simulink model "AirManagementSystem"  (R2018b)
settings: Solver=ode4  StartTime=0.0  StopTime=14400  FixedStep=dt  RelTol=1e-3
values from neighbouring files (symbols this model uses):
  AirSourceMode = 2    [run_sim.m]
  dt = 0.01    [run_sim.m]    (also in sys_id_pipeline.m = mean(diff(Time_vec_full)))
  K31 = Result31.K_slope    [sys_id_pipeline.m]
  K32 = Result32.K_slope    [sys_id_pipeline.m]
  P_ref = GlobalParams.P_ref    [sys_id_pipeline.m]
  Patm = GlobalParams.Patm    [sys_id_pipeline.m]
  R_gas = GlobalParams.R    [sys_id_pipeline.m]
  T_ref = GlobalParams.T_ref    [sys_id_pipeline.m]
  Tau31 = 5    [sys_id_pipeline.m]
  Tau32 = 5    [sys_id_pipeline.m]
  Tp31 = Result31.Tp    [sys_id_pipeline.m]
  Tp32 = Result32.Tp    [sys_id_pipeline.m]
  V_vol = pi * (0.05)^2 * 5    (= 0.0392699081699)    [run_sim.m]
  X31_den = sys_X31.Denominator    [sys_id_value.m]
  X31_num = sys_X31.Numerator    [sys_id_value.m]
  X32_den = sys_X32.Denominator    [sys_id_value.m]
  X32_num = sys_X32.Numerator    [sys_id_value.m]
libraries: simulink x8
(part 1 of 2)
settings Model: Creator=ZhaoJiance  LastModifiedBy=ZhaoJiance

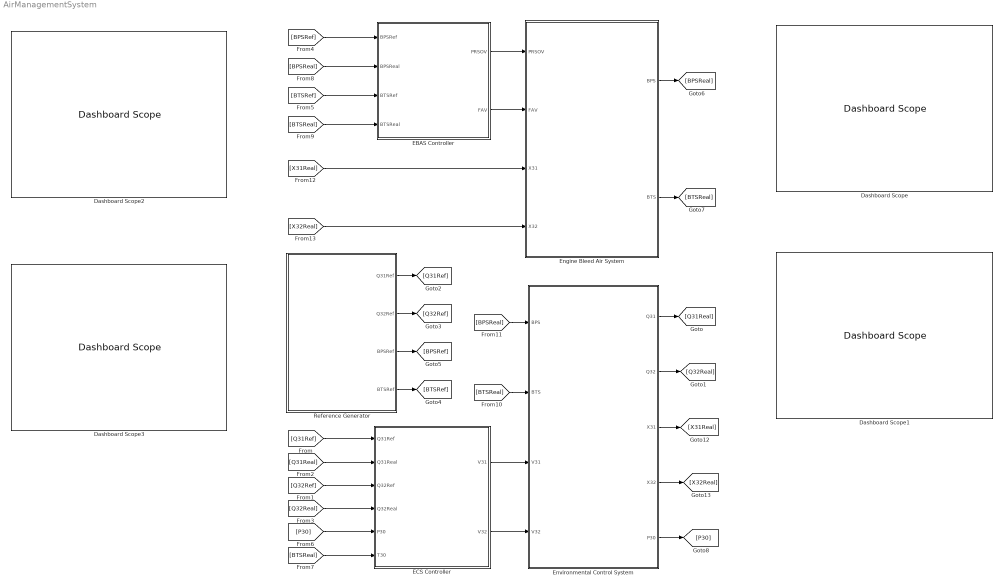
== system AirManagementSystem ==
  Dashboard Scope : DashboardScope  WebBlockId=509
  Dashboard Scope1 : DashboardScope  WebBlockId=510
  Dashboard Scope2 : DashboardScope  WebBlockId=511
  Dashboard Scope3 : DashboardScope  WebBlockId=512
  EBAS Controller : Subsystem  VariantControlMode=Label  Variant=on  VariantControl=Variant1  LabelModeActiveChoice=ASMC
  ECS Controller : Subsystem  VariantControlMode=Label  Variant=on  VariantControl=Variant1  LabelModeActiveChoice=Smith_PI_Controller
  Engine Bleed Air System : Subsystem
  Environmental Control System : Subsystem
  Reference Generator : Subsystem
  wires:
  Environmental Control System/1(Q31) -> [Q31Real]
  Environmental Control System/2(Q32) -> [Q32Real]
  [Q31Ref] -> ECS Controller/1("Q31Ref ")
  [Q31Real] -> ECS Controller/2("Q31Real ")
  [Q32Ref] -> ECS Controller/3("Q32Ref ")
  [Q32Real] -> ECS Controller/4("Q32Real ")
  [P30] -> ECS Controller/5("P30 ")
  [BTSReal] -> ECS Controller/6("T30 ")
  ECS Controller/1(" V31") -> Environmental Control System/3(V31)
  ECS Controller/2(" V32") -> Environmental Control System/4(V32)
  [BPSReal] -> Environmental Control System/1(BPS)
  [BTSReal] -> Environmental Control System/2(BTS)
  Environmental Control System/4(X32) -> [X32Real]
  Environmental Control System/3(X31) -> [X31Real]
  Reference Generator/3(BPSRef) -> [BPSRef]
  EBAS Controller/1(" PRSOV") -> Engine Bleed Air System/1(PRSOV)
  Reference Generator/2(Q32Ref) -> [Q32Ref]
  Engine Bleed Air System/2(BTS) -> [BTSReal]
  Reference Generator/1(Q31Ref) -> [Q31Ref]
  [BTSReal] -> EBAS Controller/4("BTSReal  ")
  [BPSRef] -> EBAS Controller/1("BPSRef  ")
  Engine Bleed Air System/1(BPS) -> [BPSReal]
  [BTSRef] -> EBAS Controller/3("BTSRef  ")
  EBAS Controller/2(" FAV") -> Engine Bleed Air System/2(FAV)
  [BPSReal] -> EBAS Controller/2("BPSReal ")
  Reference Generator/4(BTSRef) -> [BTSRef]
  [X31Real] -> Engine Bleed Air System/3(X31)
  [X32Real] -> Engine Bleed Air System/4(X32)
  Environmental Control System/5(P30) -> [P30]

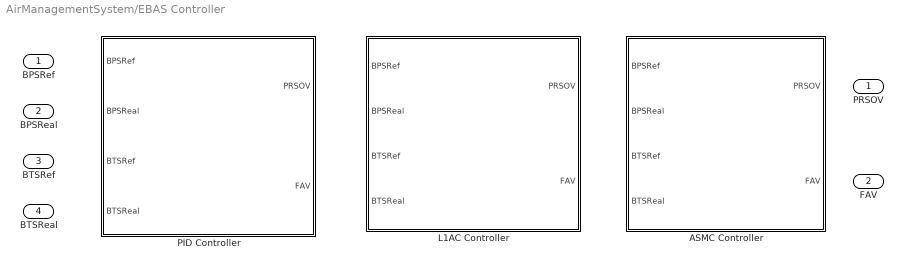
== system AirManagementSystem/EBAS Controller ==
  "BPSRef  " : Inport
  "BPSReal " : Inport  Port=2
  "BTSRef  " : Inport  Port=3
  "BTSReal  " : Inport  Port=4
  ASMC Controller : Subsystem  VariantControl=ASMC
  L1AC Controller : Subsystem  VariantControl=L1AC
  PID Controller : Subsystem  VariantControl=PID
  " PRSOV" : Outport
  " FAV" : Outport  Port=2

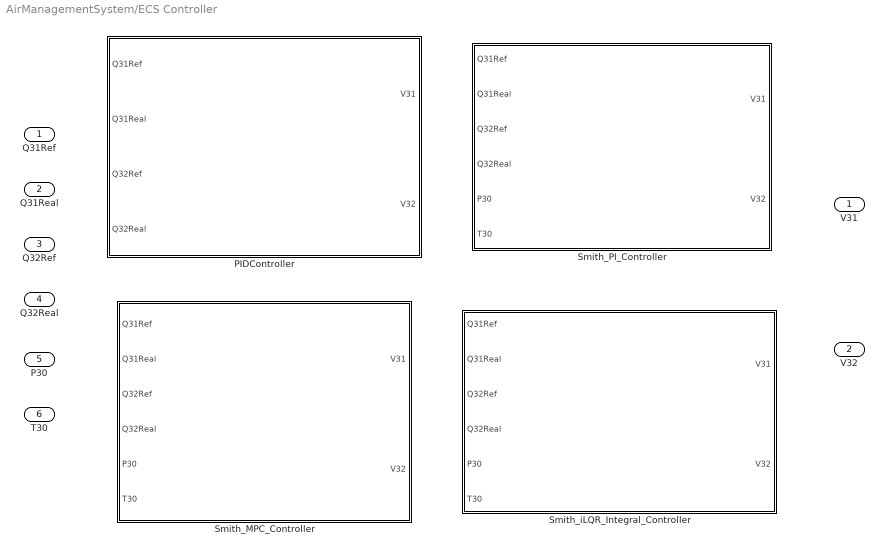
== system AirManagementSystem/ECS Controller ==
  "Q31Ref " : Inport
  "Q31Real " : Inport  Port=2
  "Q32Ref " : Inport  Port=3
  "Q32Real " : Inport  Port=4
  "P30 " : Inport  Port=5
  "T30 " : Inport  Port=6
  PIDController : Subsystem  VariantControl=PID
  Smith_MPC_Controller : Subsystem  VariantControl=Smith_MPC_Controller
  Smith_PI_Controller : Subsystem  VariantControl=Smith_PI_Controller
  Smith_iLQR_Integral_Controller : Subsystem  VariantControl=Variant
  " V31" : Outport
  " V32" : Outport  Port=2

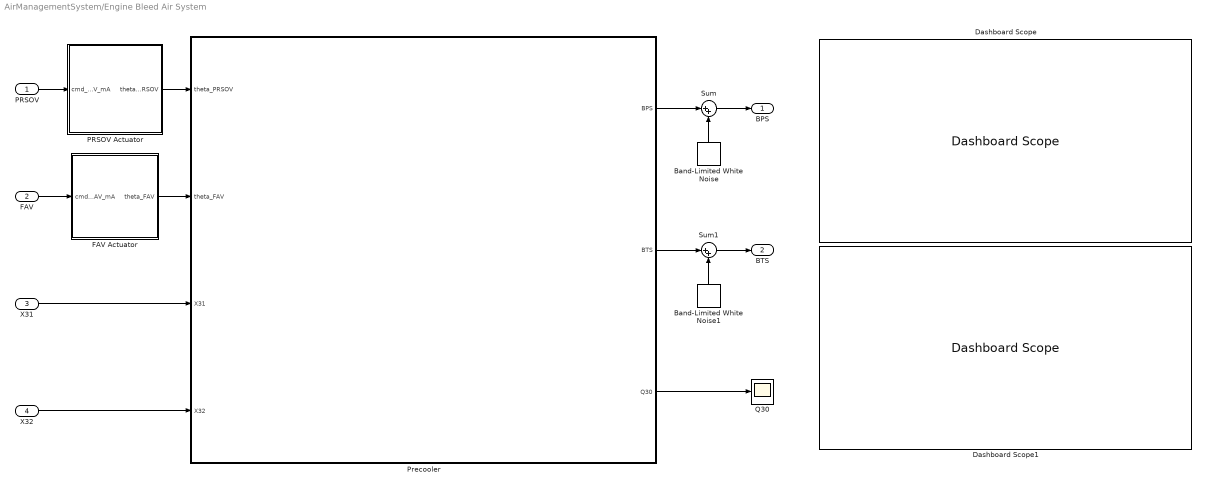
== system AirManagementSystem/Engine Bleed Air System ==
  PRSOV : Inport
  FAV : Inport  Port=2
  X31 : Inport  Port=3
  X32 : Inport  Port=4
  Band-Limited White Noise : simulink/Sources/Band-Limited White Noise  Cov=Knoise  Ts=dt  seed=[23341]
  Band-Limited White Noise1 : simulink/Sources/Band-Limited White Noise  Cov=Knoise  Ts=dt  seed=[23341]
  Dashboard Scope : DashboardScope  WebBlockId=669
  Dashboard Scope1 : DashboardScope  WebBlockId=670
  FAV Actuator : MATLAB Function  TreatAsAtomicUnit=on  SystemSampleTime=dt
  PRSOV Actuator : MATLAB Function  TreatAsAtomicUnit=on  SystemSampleTime=dt
  Precooler : Subsystem
      mask Display: image('C:\Users\ZhaoJiance\Documents\Github\AeroBleedSimulation\SysID\figure\Precooler.png');
  Q30 : Scope
  Sum : Sum  Inputs=|++
  Sum1 : Sum  Inputs=|++
  BPS : Outport
  BTS : Outport  Port=2
  wires:
  FAV/1 -> FAV Actuator/1(cmd_FAV_mA)
  PRSOV/1 -> PRSOV Actuator/1(cmd_PRSOV_mA)
  PRSOV Actuator/1(theta_PRSOV) -> Precooler/1(theta_PRSOV)
  FAV Actuator/1(theta_FAV) -> Precooler/2(theta_FAV)
  Precooler/3(Q30) -> Q30/1
  X31/1 -> Precooler/3(X31)
  X32/1 -> Precooler/4(X32)
  Sum/1 -> BPS/1
  Precooler/1(BPS) -> Sum/1
  Band-Limited White Noise/1 -> Sum/2
  Band-Limited White Noise1/1 -> Sum1/2
  Sum1/1 -> BTS/1
  Precooler/2(BTS) -> Sum1/1

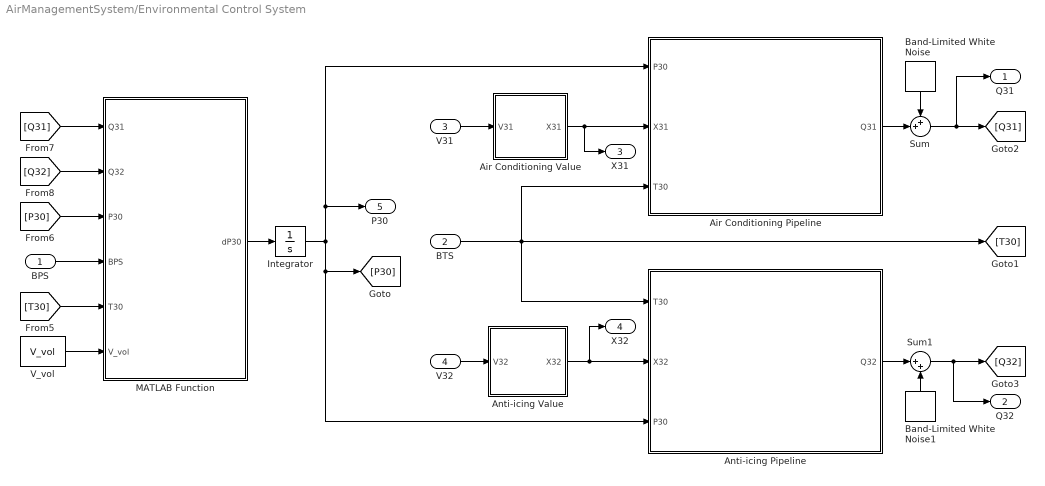
== system AirManagementSystem/Environmental Control System ==
  BPS : Inport
  BTS : Inport  Port=2
  V31 : Inport  Port=3
  V32 : Inport  Port=4
  Air Conditioning Pipeline : Subsystem
  Air Conditioning Value : Subsystem
  "Anti-icing Pipeline " : Subsystem
  Anti-icing Value : Subsystem
  Band-Limited White Noise : simulink/Sources/Band-Limited White Noise  Cov=Knoise  Ts=dt  seed=[23341]
  Band-Limited White Noise1 : simulink/Sources/Band-Limited White Noise  Cov=Knoise  Ts=dt  seed=[23341]
  Integrator : Integrator
  MATLAB Function : MATLAB Function  TreatAsAtomicUnit=on  SystemSampleTime=dt
  Sum : Sum  Inputs=++|
  Sum1 : Sum  Inputs=|++
  V_vol : Constant  Value=V_vol
  Q31 : Outport
  Q32 : Outport  Port=2
  X31 : Outport  Port=3
  X32 : Outport  Port=4
  P30 : Outport  Port=5
  wires:
  Air Conditioning Value/1(X31) -> X31/1, Air Conditioning Pipeline/2(X31)
  BPS/1 -> MATLAB Function/4(BPS)
  Integrator/1 -> Air Conditioning Pipeline/1(P30), P30/1, "Anti-icing Pipeline "/3(P30), [P30]
  Anti-icing Value/1(X32) -> X32/1, "Anti-icing Pipeline "/2(X32)
  V31/1 -> Air Conditioning Value/1(V31)
  MATLAB Function/1(dP30) -> Integrator/1
  [Q32] -> MATLAB Function/2(Q32)
  [Q31] -> MATLAB Function/1(Q31)
  V_vol/1 -> MATLAB Function/6(V_vol)
  [P30] -> MATLAB Function/3(P30)
  [T30] -> MATLAB Function/5(T30)
  V32/1 -> Anti-icing Value/1(V32)
  BTS/1 -> [T30], "Anti-icing Pipeline "/1(T30), Air Conditioning Pipeline/3(T30)
  Sum/1 -> [Q31], Q31/1
  Sum1/1 -> Q32/1, [Q32]
  "Anti-icing Pipeline "/1(Q32) -> Sum1/1
  Air Conditioning Pipeline/1(Q31) -> Sum/2
  Band-Limited White Noise/1 -> Sum/1
  Band-Limited White Noise1/1 -> Sum1/2

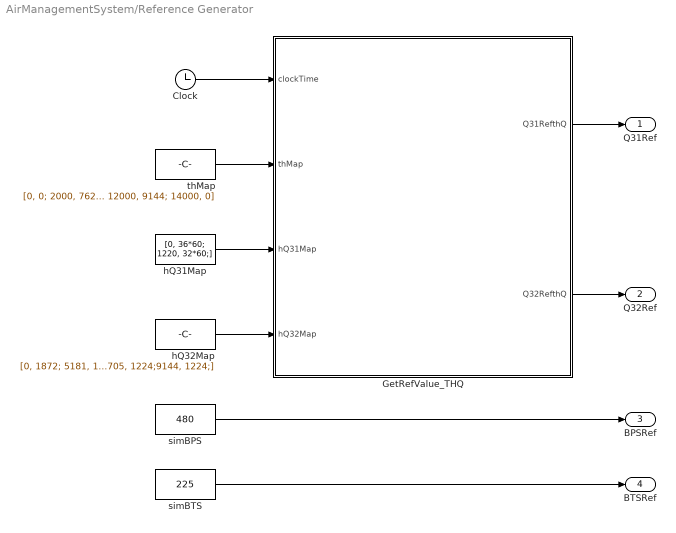
== system AirManagementSystem/Reference Generator ==
  Clock : Clock
  GetRefValue_THQ : MATLAB Function  TreatAsAtomicUnit=on  SystemSampleTime=dt
  hQ31Map : Constant  Value=[0, 36*60; 1220, 32*60;]
  hQ32Map : Constant  Value=[0, 1872; 5181, 1872; 6705, 1224;9144, 1224;]
  simBPS : Constant  Value=480
  simBTS : Constant  Value=225
  thMap : Constant  Value=[0, 0; 2000, 7620; 4000, 7620;6000, 12192; 8000, 12192; 10000, 9144; 12000, 9144; 14000, 0]
  Q31Ref : Outport
  Q32Ref : Outport  Port=2
  BPSRef : Outport  Port=3
  BTSRef : Outport  Port=4
  wires:
  Clock/1 -> GetRefValue_THQ/1(clockTime)
  thMap/1 -> GetRefValue_THQ/2(thMap)
  hQ31Map/1 -> GetRefValue_THQ/3(hQ31Map)
  GetRefValue_THQ/1(Q31RefthQ) -> Q31Ref/1
  hQ32Map/1 -> GetRefValue_THQ/4(hQ32Map)
  GetRefValue_THQ/2(Q32RefthQ) -> Q32Ref/1
  simBTS/1 -> BTSRef/1
  simBPS/1 -> BPSRef/1

== system AirManagementSystem/EBAS Controller/ASMC Controller ==
  "BPSRef  " : Inport
  "BPSReal " : Inport  Port=2
  "BTSRef  " : Inport  Port=3
  "BTSReal  " : Inport  Port=4
  ASMCController : MATLAB Function  TreatAsAtomicUnit=on  SystemSampleTime=dt
  " PRSOV" : Outport
  " FAV" : Outport  Port=2
  wires:
  ASMCController/1(PRSOV) -> " PRSOV"/1
  ASMCController/2(FAV) -> " FAV"/1
  "BPSRef  "/1 -> ASMCController/1(BPSRef)
  "BPSReal "/1 -> ASMCController/2(BPSReal)
  "BTSRef  "/1 -> ASMCController/3(BTSRef)
  "BTSReal  "/1 -> ASMCController/4(BTSReal)

== system AirManagementSystem/EBAS Controller/L1AC Controller ==
  "BPSRef  " : Inport
  "BPSReal " : Inport  Port=2
  "BTSRef  " : Inport  Port=3
  "BTSReal  " : Inport  Port=4
  FAV L1AC Controller : MATLAB Function  TreatAsAtomicUnit=on
  PRSOV L1AC Controller : MATLAB Function  TreatAsAtomicUnit=on
  " PRSOV" : Outport
  " FAV" : Outport  Port=2
  wires:
  FAV L1AC Controller/1(u_cmd) -> " FAV"/1
  PRSOV L1AC Controller/1(u_cmd) -> " PRSOV"/1
  "BPSRef  "/1 -> PRSOV L1AC Controller/1(Target)
  "BPSReal "/1 -> PRSOV L1AC Controller/2(Measured)
  "BTSReal  "/1 -> FAV L1AC Controller/2(Measured)
  "BTSRef  "/1 -> FAV L1AC Controller/1(Target)

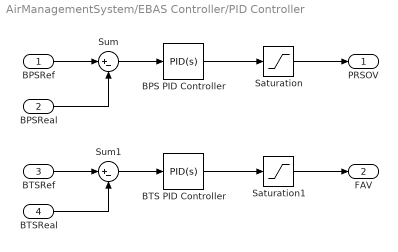
== system AirManagementSystem/EBAS Controller/PID Controller ==
  "BPSRef " : Inport
  BPSReal : Inport  Port=2
  "BTSRef " : Inport  Port=3
  "BTSReal " : Inport  Port=4
  BPS PID Controller : simulink/Continuous/PID Controller  Controller=PID  Form=Parallel  TimeDomain=Continuous-time  SampleTime=-1  IntegratorMethod=Forward Euler  FilterMethod=Forward Euler  ControllerParametersSource=internal  P=0.1  I=0.2  D=0.01  UseFilter=on  N=100  TunerSelectOption=Transfer Function Based (PID Tuner App)  InitialConditionSource=internal  InitialConditionForIntegrator=0  InitialConditionForFilter=0  DifferentiatorICPrevScaledInput=0  ExternalReset=none  TrackingMode=off  Kt=1  LimitOutput=off  UpperSaturationLimit=inf  LowerSaturationLimit=-inf  LinearizeAsGain=on  AntiWindupMode=none  Kb=1  POutMin=[]  POutMax=[]  IOutMin=[]  IOutMax=[]  DOutMin=[]  DOutMax=[]  NOutMin=[]  NOutMax=[]  SumOutMin=[]  SumOutMax=[]  SaturationOutMin=[]  SaturationOutMax=[]  PParamMin=[]  PParamMax=[]  IParamMin=[]  IParamMax=[]  DParamMin=[]  DParamMax=[]  NParamMin=[]  NParamMax=[]  KbParamMin=[]  KbParamMax=[]  KtParamMin=[]  KtParamMax=[]  KbOutMin=[]  KbOutMax=[]  KtOutMin=[]  KtOutMax=[]  IntegratorOutMin=[]  IntegratorOutMax=[]  FilterOutMin=[]  FilterOutMax=[]  SumI1OutMin=[]  SumI1OutMax=[]  SumI2OutMin=[]  SumI2OutMax=[]  SumI3OutMin=[]  SumI3OutMax=[]  SumI4OutMin=[]  SumI4OutMax=[]  SumDOutMin=[]  SumDOutMax=[]  DifferentiatorOutMin=[]  DifferentiatorOutMax=[]  FilterDiffOutCoefMin=[]  FilterDiffOutCoefMax=[]  ReciprocalOutMin=[]  ReciprocalOutMax=[]  SumDenOutMin=[]  SumDenOutMax=[]  SumNumOutMin=[]  SumNumOutMax=[]  DivideOutMin=[]  DivideOutMax=[]  IntegratorContinuousStateAttributes=''  IntegratorStateMustResolveToSignalObject=off  IntegratorRTWStateStorageClass=Auto  FilterContinuousStateAttributes=''  FilterStateMustResolveToSignalObject=off  FilterRTWStateStorageClass=Auto  ParallelPVariant=InternalParameters  IdealPVariant=Disabled  IVariant=InternalParameters  DVariant=InternalParameters  IntegratorVariant=Continuous  SatVariant=Disabled  AWVariant=Passthrough  PCopyVariant=Disabled  TRVariant=Disabled  FdbkBlocksVariant=Forward  IdealPFdbkVariant=Disabled  SatFdbkVariant=Disabled  DerivativeFilterVariant=ContFilter  NVariant=InternalParameters  NCopyVariant=Disabled  FilterICVariant=InternalICsFilter  IntegratorICVariant=InternalICs  ExternalResetVariant=Disabled  TRSumVariant=Passthrough  SumFdbkVariant=Disabled  SumVariant=Sum_PID
  BTS PID Controller : simulink/Continuous/PID Controller  Controller=PID  Form=Parallel  TimeDomain=Continuous-time  SampleTime=-1  IntegratorMethod=Forward Euler  FilterMethod=Forward Euler  ControllerParametersSource=internal  P=-0.1  I=-0.15  D=0  UseFilter=on  N=100  TunerSelectOption=Transfer Function Based (PID Tuner App)  InitialConditionSource=internal  InitialConditionForIntegrator=0  InitialConditionForFilter=0  DifferentiatorICPrevScaledInput=0  ExternalReset=none  TrackingMode=off  Kt=1  LimitOutput=off  UpperSaturationLimit=inf  LowerSaturationLimit=-inf  LinearizeAsGain=on  AntiWindupMode=none  Kb=1  POutMin=[]  POutMax=[]  IOutMin=[]  IOutMax=[]  DOutMin=[]  DOutMax=[]  NOutMin=[]  NOutMax=[]  SumOutMin=[]  SumOutMax=[]  SaturationOutMin=[]  SaturationOutMax=[]  PParamMin=[]  PParamMax=[]  IParamMin=[]  IParamMax=[]  DParamMin=[]  DParamMax=[]  NParamMin=[]  NParamMax=[]  KbParamMin=[]  KbParamMax=[]  KtParamMin=[]  KtParamMax=[]  KbOutMin=[]  KbOutMax=[]  KtOutMin=[]  KtOutMax=[]  IntegratorOutMin=[]  IntegratorOutMax=[]  FilterOutMin=[]  FilterOutMax=[]  SumI1OutMin=[]  SumI1OutMax=[]  SumI2OutMin=[]  SumI2OutMax=[]  SumI3OutMin=[]  SumI3OutMax=[]  SumI4OutMin=[]  SumI4OutMax=[]  SumDOutMin=[]  SumDOutMax=[]  DifferentiatorOutMin=[]  DifferentiatorOutMax=[]  FilterDiffOutCoefMin=[]  FilterDiffOutCoefMax=[]  ReciprocalOutMin=[]  ReciprocalOutMax=[]  SumDenOutMin=[]  SumDenOutMax=[]  SumNumOutMin=[]  SumNumOutMax=[]  DivideOutMin=[]  DivideOutMax=[]  IntegratorContinuousStateAttributes=''  IntegratorStateMustResolveToSignalObject=off  IntegratorRTWStateStorageClass=Auto  FilterContinuousStateAttributes=''  FilterStateMustResolveToSignalObject=off  FilterRTWStateStorageClass=Auto  ParallelPVariant=InternalParameters  IdealPVariant=Disabled  IVariant=InternalParameters  DVariant=InternalParameters  IntegratorVariant=Continuous  SatVariant=Disabled  AWVariant=Passthrough  PCopyVariant=Disabled  TRVariant=Disabled  FdbkBlocksVariant=Forward  IdealPFdbkVariant=Disabled  SatFdbkVariant=Disabled  DerivativeFilterVariant=ContFilter  NVariant=InternalParameters  NCopyVariant=Disabled  FilterICVariant=InternalICsFilter  IntegratorICVariant=InternalICs  ExternalResetVariant=Disabled  TRSumVariant=Passthrough  SumFdbkVariant=Disabled  SumVariant=Sum_PID
  Saturation : Saturate  UpperLimit=400  LowerLimit=0
  Saturation1 : Saturate  UpperLimit=350  LowerLimit=0
  Sum : Sum  Inputs=|+-
  Sum1 : Sum  Inputs=|+-
  PRSOV : Outport
  FAV : Outport  Port=2
  wires:
  Sum1/1 -> BTS PID Controller/1
  BPS PID Controller/1 -> Saturation/1
  BTS PID Controller/1 -> Saturation1/1
  Sum/1 -> BPS PID Controller/1
  BPSReal/1 -> Sum/2
  "BPSRef "/1 -> Sum/1
  "BTSReal "/1 -> Sum1/2
  "BTSRef "/1 -> Sum1/1
  Saturation/1 -> PRSOV/1
  Saturation1/1 -> FAV/1

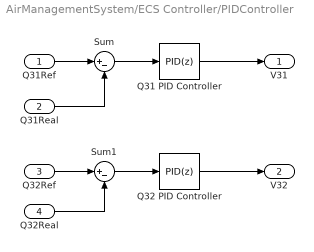
== system AirManagementSystem/ECS Controller/PIDController ==
  Q31Ref : Inport
  Q31Real : Inport  Port=2
  Q32Ref : Inport  Port=3
  Q32Real : Inport  Port=4
  Q31 PID Controller : simulink/Continuous/PID Controller  Controller=PID  Form=Parallel  TimeDomain=Discrete-time  SampleTime=-1  IntegratorMethod=Forward Euler  FilterMethod=Forward Euler  ControllerParametersSource=internal  P=0.0332634866006577  I=0.00162963841502539  D=0.0693776015925971  UseFilter=on  N=0.140831158638555  TunerSelectOption=Transfer Function Based (PID Tuner App)  InitialConditionSource=internal  InitialConditionForIntegrator=0  InitialConditionForFilter=0  DifferentiatorICPrevScaledInput=0  ExternalReset=none  TrackingMode=off  Kt=1  LimitOutput=off  UpperSaturationLimit=inf  LowerSaturationLimit=-inf  LinearizeAsGain=on  AntiWindupMode=none  Kb=1  POutMin=[]  POutMax=[]  IOutMin=[]  IOutMax=[]  DOutMin=[]  DOutMax=[]  NOutMin=[]  NOutMax=[]  SumOutMin=[]  SumOutMax=[]  SaturationOutMin=[]  SaturationOutMax=[]  PParamMin=[]  PParamMax=[]  IParamMin=[]  IParamMax=[]  DParamMin=[]  DParamMax=[]  NParamMin=[]  NParamMax=[]  KbParamMin=[]  KbParamMax=[]  KtParamMin=[]  KtParamMax=[]  KbOutMin=[]  KbOutMax=[]  KtOutMin=[]  KtOutMax=[]  IntegratorOutMin=[]  IntegratorOutMax=[]  FilterOutMin=[]  FilterOutMax=[]  SumI1OutMin=[]  SumI1OutMax=[]  SumI2OutMin=[]  SumI2OutMax=[]  SumI3OutMin=[]  SumI3OutMax=[]  SumI4OutMin=[]  SumI4OutMax=[]  SumDOutMin=[]  SumDOutMax=[]  DifferentiatorOutMin=[]  DifferentiatorOutMax=[]  FilterDiffOutCoefMin=[]  FilterDiffOutCoefMax=[]  ReciprocalOutMin=[]  ReciprocalOutMax=[]  SumDenOutMin=[]  SumDenOutMax=[]  SumNumOutMin=[]  SumNumOutMax=[]  DivideOutMin=[]  DivideOutMax=[]  IntegratorContinuousStateAttributes=''  IntegratorStateMustResolveToSignalObject=off  IntegratorRTWStateStorageClass=Auto  FilterContinuousStateAttributes=''  FilterStateMustResolveToSignalObject=off  FilterRTWStateStorageClass=Auto  ParallelPVariant=InternalParameters  IdealPVariant=Disabled  IVariant=InternalParameters  DVariant=InternalParameters  IntegratorVariant=Discrete  SatVariant=Disabled  AWVariant=Passthrough  PCopyVariant=Disabled  TRVariant=Disabled  FdbkBlocksVariant=Forward  IdealPFdbkVariant=Disabled  SatFdbkVariant=Disabled  DerivativeFilterVariant=ForwardEulerFilter  NVariant=InternalParameters  NCopyVariant=Disabled  FilterICVariant=InternalICsFilter  IntegratorICVariant=InternalICs  ExternalResetVariant=Disabled  TRSumVariant=Passthrough  SumFdbkVariant=Disabled  SumVariant=Sum_PID
  Q32 PID Controller : simulink/Continuous/PID Controller  Controller=PID  Form=Parallel  TimeDomain=Discrete-time  SampleTime=-1  IntegratorMethod=Forward Euler  FilterMethod=Forward Euler  ControllerParametersSource=internal  P=0.0550164924963942  I=0.00248684748202474  D=0.0884119468512251  UseFilter=on  N=14.1148734165854  TunerSelectOption=Transfer Function Based (PID Tuner App)  InitialConditionSource=internal  InitialConditionForIntegrator=0  InitialConditionForFilter=0  DifferentiatorICPrevScaledInput=0  ExternalReset=none  TrackingMode=off  Kt=1  LimitOutput=off  UpperSaturationLimit=inf  LowerSaturationLimit=-inf  LinearizeAsGain=on  AntiWindupMode=none  Kb=1  POutMin=[]  POutMax=[]  IOutMin=[]  IOutMax=[]  DOutMin=[]  DOutMax=[]  NOutMin=[]  NOutMax=[]  SumOutMin=[]  SumOutMax=[]  SaturationOutMin=[]  SaturationOutMax=[]  PParamMin=[]  PParamMax=[]  IParamMin=[]  IParamMax=[]  DParamMin=[]  DParamMax=[]  NParamMin=[]  NParamMax=[]  KbParamMin=[]  KbParamMax=[]  KtParamMin=[]  KtParamMax=[]  KbOutMin=[]  KbOutMax=[]  KtOutMin=[]  KtOutMax=[]  IntegratorOutMin=[]  IntegratorOutMax=[]  FilterOutMin=[]  FilterOutMax=[]  SumI1OutMin=[]  SumI1OutMax=[]  SumI2OutMin=[]  SumI2OutMax=[]  SumI3OutMin=[]  SumI3OutMax=[]  SumI4OutMin=[]  SumI4OutMax=[]  SumDOutMin=[]  SumDOutMax=[]  DifferentiatorOutMin=[]  DifferentiatorOutMax=[]  FilterDiffOutCoefMin=[]  FilterDiffOutCoefMax=[]  ReciprocalOutMin=[]  ReciprocalOutMax=[]  SumDenOutMin=[]  SumDenOutMax=[]  SumNumOutMin=[]  SumNumOutMax=[]  DivideOutMin=[]  DivideOutMax=[]  IntegratorContinuousStateAttributes=''  IntegratorStateMustResolveToSignalObject=off  IntegratorRTWStateStorageClass=Auto  FilterContinuousStateAttributes=''  FilterStateMustResolveToSignalObject=off  FilterRTWStateStorageClass=Auto  ParallelPVariant=InternalParameters  IdealPVariant=Disabled  IVariant=InternalParameters  DVariant=InternalParameters  IntegratorVariant=Discrete  SatVariant=Disabled  AWVariant=Passthrough  PCopyVariant=Disabled  TRVariant=Disabled  FdbkBlocksVariant=Forward  IdealPFdbkVariant=Disabled  SatFdbkVariant=Disabled  DerivativeFilterVariant=ForwardEulerFilter  NVariant=InternalParameters  NCopyVariant=Disabled  FilterICVariant=InternalICsFilter  IntegratorICVariant=InternalICs  ExternalResetVariant=Disabled  TRSumVariant=Passthrough  SumFdbkVariant=Disabled  SumVariant=Sum_PID
  Sum : Sum  Inputs=|+-
  Sum1 : Sum  Inputs=|+-
  V31 : Outport
  V32 : Outport  Port=2
  wires:
  Q31Ref/1 -> Sum/1
  Sum/1 -> Q31 PID Controller/1
  Q32Real/1 -> Sum1/2
  Q32Ref/1 -> Sum1/1
  Q31Real/1 -> Sum/2
  Q31 PID Controller/1 -> V31/1
  Q32 PID Controller/1 -> V32/1
  Sum1/1 -> Q32 PID Controller/1

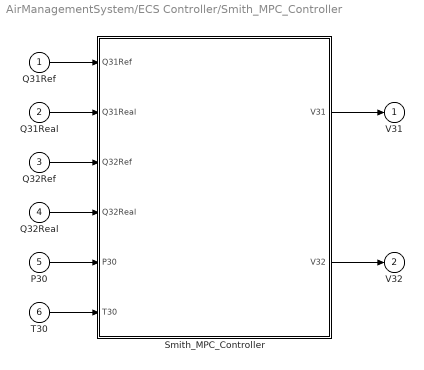
== system AirManagementSystem/ECS Controller/Smith_MPC_Controller ==
  "Q31Ref " : Inport
  "Q31Real " : Inport  Port=2
  "Q32Ref " : Inport  Port=3
  "Q32Real " : Inport  Port=4
  "P30 " : Inport  Port=5
  "T30 " : Inport  Port=6
  Smith_MPC_Controller : MATLAB Function  TreatAsAtomicUnit=on
  " V31" : Outport
  " V32" : Outport  Port=2
  wires:
  "Q31Ref "/1 -> Smith_MPC_Controller/1(Q31Ref)
  "Q31Real "/1 -> Smith_MPC_Controller/2(Q31Real)
  "T30 "/1 -> Smith_MPC_Controller/6(T30)
  "P30 "/1 -> Smith_MPC_Controller/5(P30)
  "Q32Real "/1 -> Smith_MPC_Controller/4(Q32Real)
  "Q32Ref "/1 -> Smith_MPC_Controller/3(Q32Ref)
  Smith_MPC_Controller/2(V32) -> " V32"/1
  Smith_MPC_Controller/1(V31) -> " V31"/1

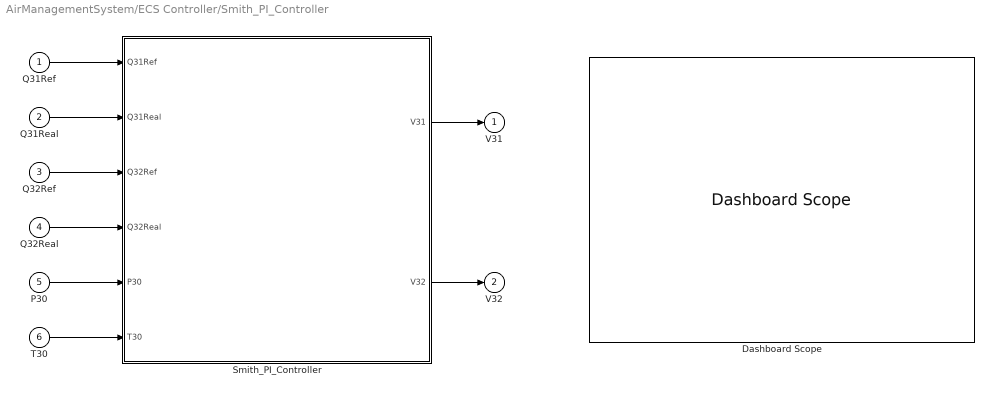
== system AirManagementSystem/ECS Controller/Smith_PI_Controller ==
  "Q31Ref " : Inport
  "Q31Real " : Inport  Port=2
  "Q32Ref " : Inport  Port=3
  "Q32Real " : Inport  Port=4
  "P30 " : Inport  Port=5
  "T30 " : Inport  Port=6
  Dashboard Scope : DashboardScope  WebBlockId=940
  Smith_PI_Controller : MATLAB Function  TreatAsAtomicUnit=on
  " V31" : Outport
  " V32" : Outport  Port=2
  wires:
  Smith_PI_Controller/1(V31) -> " V31"/1
  Smith_PI_Controller/2(V32) -> " V32"/1
  "Q31Ref "/1 -> Smith_PI_Controller/1(Q31Ref)
  "Q31Real "/1 -> Smith_PI_Controller/2(Q31Real)
  "Q32Ref "/1 -> Smith_PI_Controller/3(Q32Ref)
  "Q32Real "/1 -> Smith_PI_Controller/4(Q32Real)
  "P30 "/1 -> Smith_PI_Controller/5(P30)
  "T30 "/1 -> Smith_PI_Controller/6(T30)

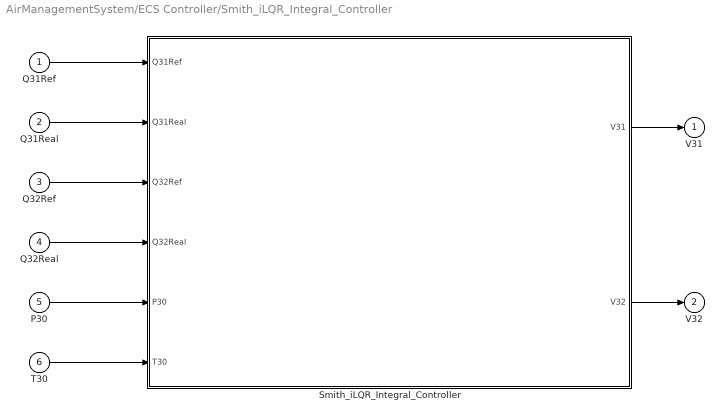
== system AirManagementSystem/ECS Controller/Smith_iLQR_Integral_Controller ==
  "Q31Ref " : Inport
  "Q31Real " : Inport  Port=2
  "Q32Ref " : Inport  Port=3
  "Q32Real " : Inport  Port=4
  "P30 " : Inport  Port=5
  "T30 " : Inport  Port=6
  Smith_iLQR_Integral_Controller : MATLAB Function  TreatAsAtomicUnit=on
  " V31" : Outport
  " V32" : Outport  Port=2
  wires:
  Smith_iLQR_Integral_Controller/1(V31) -> " V31"/1
  Smith_iLQR_Integral_Controller/2(V32) -> " V32"/1
  "Q31Real "/1 -> Smith_iLQR_Integral_Controller/2(Q31Real)
  "Q31Ref "/1 -> Smith_iLQR_Integral_Controller/1(Q31Ref)
  "Q32Ref "/1 -> Smith_iLQR_Integral_Controller/3(Q32Ref)
  "Q32Real "/1 -> Smith_iLQR_Integral_Controller/4(Q32Real)
  "P30 "/1 -> Smith_iLQR_Integral_Controller/5(P30)
  "T30 "/1 -> Smith_iLQR_Integral_Controller/6(T30)

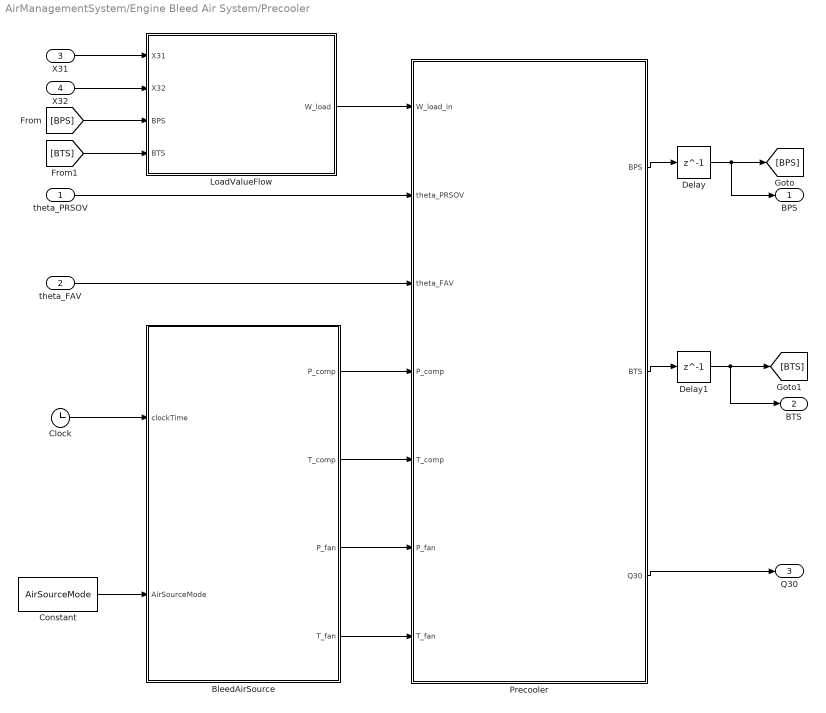
== system AirManagementSystem/Engine Bleed Air System/Precooler ==
  theta_PRSOV : Inport
  theta_FAV : Inport  Port=2
  X31 : Inport  Port=3
  X32 : Inport  Port=4
  BleedAirSource : MATLAB Function  TreatAsAtomicUnit=on  SystemSampleTime=dt
  Clock : Clock
  Constant : Constant  Value=AirSourceMode
  Delay : Delay  DelayLength=1  InitialCondition=0
  Delay1 : Delay  DelayLength=1  InitialCondition=0
  LoadValueFlow : MATLAB Function  TreatAsAtomicUnit=on  SystemSampleTime=dt
  Precooler : MATLAB Function  TreatAsAtomicUnit=on  SystemSampleTime=dt
  BPS : Outport
  BTS : Outport  Port=2
  Q30 : Outport  Port=3
  wires:
  Delay/1 -> BPS/1, [BPS]
  Delay1/1 -> BTS/1, [BTS]
  LoadValueFlow/1(W_load) -> Precooler/1(W_load_in)
  Precooler/1(BPS) -> Delay/1
  Precooler/2(BTS) -> Delay1/1
  Precooler/3(Q30) -> Q30/1
  theta_PRSOV/1 -> Precooler/2(theta_PRSOV)
  theta_FAV/1 -> Precooler/3(theta_FAV)
  X31/1 -> LoadValueFlow/1(X31)
  X32/1 -> LoadValueFlow/2(X32)
  Clock/1 -> BleedAirSource/1(clockTime)
  [BTS] -> LoadValueFlow/4(BTS)
  [BPS] -> LoadValueFlow/3(BPS)
  BleedAirSource/1(P_comp) -> Precooler/4(P_comp)
  BleedAirSource/2(T_comp) -> Precooler/5(T_comp)
  BleedAirSource/3(P_fan) -> Precooler/6(P_fan)
  BleedAirSource/4(T_fan) -> Precooler/7(T_fan)
  Constant/1 -> BleedAirSource/2(AirSourceMode)

== system AirManagementSystem/Environmental Control System/Air Conditioning Pipeline ==
  P30 : Inport
  X31 : Inport  Port=2
  T30 : Inport  Port=3
  MATLAB Function : MATLAB Function  TreatAsAtomicUnit=on  SystemSampleTime=dt
  Saturation : Saturate  UpperLimit=inf  LowerLimit=0
  Transfer Fcn : TransferFcn  Denominator=[Tp31 1]
  Transport Delay : TransportDelay  DelayTime=Tau31
  Q31 : Outport
  wires:
  Transfer Fcn/1 -> Transport Delay/1
  X31/1 -> MATLAB Function/1(X)
  MATLAB Function/1(Q_static) -> Transfer Fcn/1
  T30/1 -> MATLAB Function/3(T30)
  P30/1 -> MATLAB Function/2(P30)
  Transport Delay/1 -> Saturation/1
  Saturation/1 -> Q31/1

== system AirManagementSystem/Environmental Control System/Air Conditioning Value ==
  V31 : Inport
  V31 Saturation : Saturate  UpperLimit=100  LowerLimit=0
  X31 Deadband : MATLAB Function  TreatAsAtomicUnit=on  SystemSampleTime=dt
  X31 Saturation : Saturate  UpperLimit=100  LowerLimit=0
  X31 Value System : TransferFcn  Numerator=X31_num  Denominator=X31_den
  X31 : Outport
  wires:
  X31 Deadband/1(u_eff) -> X31 Value System/1
  X31 Saturation/1 -> X31/1, X31 Deadband/1(curPos)
  X31 Value System/1 -> X31 Saturation/1
  V31/1 -> V31 Saturation/1
  V31 Saturation/1 -> X31 Deadband/2(cmdPos)

== system AirManagementSystem/Environmental Control System/Anti-icing Pipeline  ==
  T30 : Inport
  X32 : Inport  Port=2
  P30 : Inport  Port=3
  MATLAB Function : MATLAB Function  TreatAsAtomicUnit=on  SystemSampleTime=dt
  Saturation : Saturate  UpperLimit=inf  LowerLimit=0
  Transfer Fcn : TransferFcn  Denominator=[Tp32 1]
  Transport Delay : TransportDelay  DelayTime=Tau32
  Q32 : Outport
  wires:
  P30/1 -> MATLAB Function/2(P30)
  MATLAB Function/1(Q_static) -> Transfer Fcn/1
  Transfer Fcn/1 -> Transport Delay/1
  T30/1 -> MATLAB Function/3(T30)
  Transport Delay/1 -> Saturation/1
  X32/1 -> MATLAB Function/1(X)
  Saturation/1 -> Q32/1

== system AirManagementSystem/Environmental Control System/Anti-icing Value ==
  V32 : Inport
  V32 Saturation : Saturate  UpperLimit=100  LowerLimit=0
  X32 Deadband : MATLAB Function  TreatAsAtomicUnit=on  SystemSampleTime=dt
  X32 Saturation : Saturate  UpperLimit=100  LowerLimit=0
  X32 Value System : TransferFcn  Numerator=X32_num  Denominator=X32_den
  X32 : Outport
  wires:
  V32/1 -> V32 Saturation/1
  X32 Deadband/1(u_eff) -> X32 Value System/1
  X32 Saturation/1 -> X32 Deadband/1(curPos), X32/1
  X32 Value System/1 -> X32 Saturation/1
  V32 Saturation/1 -> X32 Deadband/2(cmdPos)

== matlab function AirManagementSystem/Environmental Control System/Anti-icing Value/X32 Deadband ==
  data: curPos input; u_eff output; cmdPos input
function u_eff = fcn(curPos, cmdPos)
    % 引入持久变量来记录系统当前的状态：是在"调节中"还是"已到位"
    persistent isAdjusting
    if isempty(isAdjusting)
        isAdjusting = false;
    end

    % === 参数设置 ===
    % Start_Deadband: 启动死区（防抖阈值）。误差超过此值，开始动作。
    % 设为 3，意味着噪声在 +/-3 以内时，若系统本来是静止的，就不理会。
    Start_Deadband = 2.0; 
    
    % Stop_Deadband: 停止死区（精度阈值）。误差小于此值，才算到位。
    % 设为 0.5，意味着一旦动起来，必须修到 99.5~100.5 之间才停手。
    Stop_Deadband  = 0.5; 

    % 计算当前误差绝对值
    err = abs(cmdPos - curPos);

    % === 状态机逻辑 ===
    if isAdjusting
        % 【状态1：正在调节中】
        % 既然已经动起来了，就要追求高精度。
        % 只有当误差足够小（满足精度要求）时，才停止。
        if err <= Stop_Deadband
            isAdjusting = false; % 切换状态：认为已到位
            u_eff = curPos;      % 欺骗控制器误差为0，使其停止积分/输出
        else
            isAdjusting = true;  % 保持调节状态
            u_eff = cmdPos;      % 正常输出目标值给控制器
        end
    else
        % 【状态2：已到位/静止中】
        % 此时为了防抖，对小误差视而不见。
        % 只有当误差突然变大（超过启动阈值，比如新指令来了）时，才开始动。
        if err > Start_Deadband
            isAdjusting = true;  % 切换状态：开始调节
            u_eff = cmdPos;      % 输出目标值
        else
            isAdjusting = false; % 保持静止
            u_eff = curPos;      % 锁定当前位置，抑制抖动
        end
    end
end

== matlab function AirManagementSystem/Environmental Control System/Air Conditioning Value/X31 Deadband ==
  data: curPos input; u_eff output; cmdPos input
function u_eff = fcn(curPos, cmdPos)
    % 引入持久变量来记录系统当前的状态：是在"调节中"还是"已到位"
    persistent isAdjusting
    if isempty(isAdjusting)
        isAdjusting = false;
    end

    % === 参数设置 ===
    % Start_Deadband: 启动死区（防抖阈值）。误差超过此值，开始动作。
    % 设为 3，意味着噪声在 +/-3 以内时，若系统本来是静止的，就不理会。
    Start_Deadband = 3.0; 
    
    % Stop_Deadband: 停止死区（精度阈值）。误差小于此值，才算到位。
    % 设为 0.5，意味着一旦动起来，必须修到 99.5~100.5 之间才停手。
    Stop_Deadband  = 0.5; 

    % 计算当前误差绝对值
    err = abs(cmdPos - curPos);

    % === 状态机逻辑 ===
    if isAdjusting
        % 【状态1：正在调节中】
        % 既然已经动起来了，就要追求高精度。
        % 只有当误差足够小（满足精度要求）时，才停止。
        if err <= Stop_Deadband
            isAdjusting = false; % 切换状态：认为已到位
            u_eff = curPos;      % 欺骗控制器误差为0，使其停止积分/输出
        else
            isAdjusting = true;  % 保持调节状态
            u_eff = cmdPos;      % 正常输出目标值给控制器
        end
    else
        % 【状态2：已到位/静止中】
        % 此时为了防抖，对小误差视而不见。
        % 只有当误差突然变大（超过启动阈值，比如新指令来了）时，才开始动。
        if err > Start_Deadband
            isAdjusting = true;  % 切换状态：开始调节
            u_eff = cmdPos;      % 输出目标值
        else
            isAdjusting = false; % 保持静止
            u_eff = curPos;      % 锁定当前位置，抑制抖动
        end
    end
end

== matlab function AirManagementSystem/Environmental Control System/Air Conditioning Pipeline/MATLAB Function ==
  data: X input; Q_static output; P30 input; T30 input; K31 parameter; P_ref parameter; T_ref parameter; R_gas parameter; Patm parameter
function Q_static = StaticCalc(X, P30, T30, K31, P_ref, T_ref, R_gas, Patm)
    % 输入单位说明:
    % X: 阀门开度 (0-1 或 0-100，取决于你的K是基于什么单位)
    % P_dyn: 实时压力 (kPa)
    % T_dyn: 实时温度 (摄氏度)
    
    % --- 1. 计算标称流量 (Nominal Flow) ---
    Q_nominal = K31 * X;
    
    % --- 2. 计算实时物理因子 (Real-time Term) ---
    % 温度转开尔文
    Tk_dyn = T30 + 273.15;
    delta_P_dyn = P30 - Patm;
    Term_Dyn = sqrt(max((P30 * delta_P_dyn) / (R_gas * Tk_dyn), 0));
    
    % --- 3. 计算参考物理因子 (Reference Term - Constant) ---
    Tk_ref = T_ref + 273.15;
    delta_P_ref = P_ref - Patm;
    Term_Ref = sqrt(max((P_ref * delta_P_ref) / (R_gas * Tk_ref), 0));
    
    % --- 4. 计算最终静态流量 (修正后) ---
    if Term_Ref < 1e-6
        Ratio = 1;
    else
        Ratio = Term_Dyn / Term_Ref;
    end
    
    Q_static = Q_nominal * Ratio;
end

== matlab function AirManagementSystem/Environmental Control System/Anti-icing Pipeline /MATLAB Function ==
  data: X input; Q_static output; P30 input; T30 input; K32 parameter; P_ref parameter; T_ref parameter; R_gas parameter; Patm parameter
function Q_static = StaticCalc(X, P30, T30, K32, P_ref, T_ref, R_gas, Patm)
    % 输入单位说明:
    % X: 阀门开度 (0-1 或 0-100，取决于你的K是基于什么单位)
    % P_dyn: 实时压力 (kPa)
    % T_dyn: 实时温度 (摄氏度)
    
    % --- 1. 计算标称流量 (Nominal Flow) ---
    Q_nominal = K32 * X;
    
    % --- 2. 计算实时物理因子 (Real-time Term) ---
    % 温度转开尔文
    Tk_dyn = T30 + 273.15;
    delta_P_dyn = P30 - Patm;
    Term_Dyn = sqrt(max((P30 * delta_P_dyn) / (R_gas * Tk_dyn), 0));
    
    % --- 3. 计算参考物理因子 (Reference Term - Constant) ---
    Tk_ref = T_ref + 273.15;
    delta_P_ref = P_ref - Patm;
    Term_Ref = sqrt(max((P_ref * delta_P_ref) / (R_gas * Tk_ref), 0));
    
    % --- 4. 计算最终静态流量 (修正后) ---
    if Term_Ref < 1e-6
        Ratio = 1;
    else
        Ratio = Term_Dyn / Term_Ref;
    end
    
    Q_static = Q_nominal * Ratio;
end

== matlab function AirManagementSystem/Environmental Control System/MATLAB Function ==
  data: Q31 input; dP30 output; Q32 input; P30 input; BPS input; T30 input; V_vol input; R_gas parameter
function dP30 = PressureDynamics(Q31, Q32, P30, BPS, T30, V_vol, R_gas)
    % 输入:
    % Q31, Q32: 两个支路的实时流量 (kg/h) -> 需转换为 kg/s
    % P30: 当前公共节点压力 (kPa) -> 需转换为 Pa
    % P_source: 气源总压力 (kPa)
    % V_vol: 管汇体积 (m^3)，这是一个调试参数，实际系统为2-4m长的DN100管路
    
    % --- 单位换算 ---
    Q_out_kgs = (Q31 + Q32) / 3600; % kg/h -> kg/s
    P30_Pa = P30 * 1000;
    P_source_Pa = BPS * 1000;
    T_K = T30 + 273.15;
    
    % --- 1. 计算气源供气流量 Q_in (模拟上游特性) ---
    % 假设上游是一个大减压阀或限流孔板，流量与压差有关
    % Kv_source 是上游供气能力的系数，需要大致估算
    Kv_source = 0.005; 
    
    if P_source_Pa > P30_Pa
        % 简化的亚音速/声速流动方程
        Q_in_kgs = Kv_source * sqrt(P_source_Pa - P30_Pa);
    else
        Q_in_kgs = 0;
    end
    
    % --- 2. 容腔微分方程 (dP/dt) ---
    % 根据理想气体状态方程微分形式: dP/dt = (RT/V) * (Qin - Qout)
    % 这是一个积分环节，体现了压力的建立过程
    
    dP_dt_Pa = (R_gas * T_K / V_vol) * (Q_in_kgs - Q_out_kgs);
    
    % --- 输出 ---
    dP30 = dP_dt_Pa / 1000; % 换回 kPa/s
end

== matlab function AirManagementSystem/EBAS Controller/ASMC Controller/ASMCController ==
  data: BPSRef input; PRSOV output; BPSReal input; BTSRef input; BTSReal input; FAV output; dt parameter
function [PRSOV, FAV] = ASMCController(BPSRef, BPSReal, BTSRef, BTSReal, dt)
    % =====================================================================
    % 引气系统控制器 (ESO + ASMC + 逆迟滞补偿)
    %
    % 架构说明:
    %   1. 观测层 (ESO): 实时估计系统内部状态和未知负载扰动(Total Disturbance)
    %   2. 决策层 (ASMC): 基于扰动补偿的自适应滑模控制，计算理想阀门角度
    %   3. 补偿层 (Inverse Hys): 将理想角度映射为电流，抵消物理迟滞
    %
    % 输入:
    %   BPSRef/Real : 压力期望/反馈 [kPa]
    %   BTSRef/Real : 温度期望/反馈 [degC]
    %   dt          : 采样时间 [s]
    % 输出:
    %   PRSOV    : 热路阀电流 [0-400mA]
    %   FAV      : 冷路阀电流 [0-350mA]
    % =====================================================================

    % --- 1. 系统参数与状态存储 ---
    persistent z1_p z2_p        % 压力ESO状态: z1(压力估计), z2(总扰动)
    persistent z1_t z2_t        % 温度ESO状态: z1(温度估计), z2(总扰动)
    persistent k_asmc_p         % 压力控制器自适应增益
    persistent k_asmc_t         % 温度控制器自适应增益
    persistent last_theta_p     % 上一时刻压力阀角度(用于判断方向)
    persistent last_theta_f     % 上一时刻温度阀角度
    persistent is_init          % 初始化标志

    % --- 2. 参数初始化 ---
    if isempty(is_init)
        % ESO 初始状态
        z1_p = BPSReal; z2_p = 0;
        z1_t = BTSReal; z2_t = 0;
        
        % ASMC 初始增益
        k_asmc_p = 5.0; 
        k_asmc_t = 2.0;
        
        last_theta_p = 0;
        last_theta_f = 0;
        is_init = 1;
    end

    % =====================================================================
    % 3. 压力控制回路 (Pressure Control Loop)
    %    目标: BPS -> BPSRef
    %    策略: ESO 估计负载扰动 -> ASMC 计算角度 -> 逆模型输出电流
    % =====================================================================
    
    % --- 3.1 扩张状态观测器 (ESO) ---
    % 标称控制增益 b0_p (估算值: 阀门对压力的影响率)
    % 物理意义: 开度增加1度，压力大约增加多少kPa/s
    b0_p = 20.0; 
    
    % ESO 参数 (带宽配置)
    beta1_p = 100; % 状态观测增益
    beta2_p = 100; % 扰动观测增益
    
    % 观测器误差
    e_eso_p = z1_p - BPSReal;
    
    % ESO 状态更新 (离散化欧拉法)
    % u_last 近似为上一时刻的角度 last_theta_p
    dz1_p = z2_p + b0_p * (last_theta_p/90.0) - beta1_p * e_eso_p;
    dz2_p = -beta2_p * e_eso_p;
    
    % z2_p 即为估计出的"总扰动" (包含 X31/X32 动作引起的压力跌落)
    z1_p = z1_p + dz1_p * dt;
    z2_p = z2_p + dz2_p * dt;
    
    % --- 3.2 自适应滑模控制器 (ASMC) ---
    e_p = BPSRef - BPSReal; % 跟踪误差
    
    % 自适应律: 根据误差大小调整增益
    % 误差大 -> 增益增大; 误差小 -> 增益保持
    eta_p = 2.0;
    dk_p = eta_p * abs(e_p);
    k_asmc_p = min(max(k_asmc_p + dk_p * dt, 1.0), 50.0); % 增益限幅
    
    % 控制律计算
    % u = (1/b0) * (dot_ref - z2 + k * tanh(s))
    % 这里忽略 dot_ref (假设阶跃输入)，引入 tanh 平滑切换
    phi_p = 25.0; % 边界层厚度
    u_ideal_p_norm = (1/b0_p) * (-z2_p + k_asmc_p * tanh(e_p/phi_p));
    
    % 反归一化到角度 [0, 90]
    theta_p_des = u_ideal_p_norm * 90.0;
    theta_p_des = max(0, min(90, theta_p_des)); % 物理限幅
    
    % --- 3.3 迟滞补偿 (逆模型层) ---
    % 使用查表法代替神经网络 (功能等效: 映射 理想角度 -> 实际电流)
    I_axis_P = [0, 120.0, 137.5, 155.0, 172.5, 190.0, 225.0, 260.0, 295.0, 330.0, 365.0, 400.0];
    
    Ang_Rise_P = [-1.0, 0, 3, 7, 15, 25, 45, 62, 75, 85, 89, 90]; 
    Ang_Fall_P = [-1.0, 0, 10, 25, 40, 55, 75, 85, 89, 90, 90.1, 90.2];
    
    % 判断运动方向
    if theta_p_des >= last_theta_p
        PRSOV = interp1(Ang_Rise_P, I_axis_P, theta_p_des, 'linear', 'extrap');
    else
        PRSOV = interp1(Ang_Fall_P, I_axis_P, theta_p_des, 'linear', 'extrap');
    end
    PRSOV = max(0, min(400, PRSOV));
    
    % =====================================================================
    % 4. 温度控制回路 (Temperature Control Loop)
    %    目标: BTS -> BTSRef
    %    注意: 这是一个反向响应系统 (开大冷风阀 -> 温度降低)
    % =====================================================================
    
    % --- 4.1 ESO ---
    b0_t = -10.0; % 负增益: 角度增加，温度下降
    beta1_t = 50; 
    beta2_t = 200;
    
    e_eso_t = z1_t - BTSReal;
    dz1_t = z2_t + b0_t * (last_theta_f/90.0) - beta1_t * e_eso_t;
    dz2_t = -beta2_t * e_eso_t;
    
    z1_t = z1_t + dz1_t * dt;
    z2_t = z2_t + dz2_t * dt;
    
    % --- 4.2 ASMC ---
    e_t = BTSRef - BTSReal;
    
    eta_t = 1.0;
    dk_t = eta_t * abs(e_t);
    k_asmc_t = min(max(k_asmc_t + dk_t * dt, 1.0), 30.0);
    
    % 控制律 (注意 b0_t 是负数，会自动处理方向)
    phi_t = 30;
    u_ideal_t_norm = (1/b0_t) * (-z2_t + k_asmc_t * tanh(e_t/phi_t));
    
    theta_f_des = u_ideal_t_norm * 90.0;
    theta_f_des = max(0, min(90, theta_f_des));
    
    % --- 4.3 迟滞补偿 ---
    I_axis_F = [0, 120.0000, 134.3750, 148.7500, 163.1250, 177.5000, ...
                206.2500, 235.0000, 263.7500, 292.5000, 321.2500, 350.0000];
    
    Ang_Rise_F = [-1.0, 0, 3, 7, 15, 25, 45, 62, 75, 85, 89, 90]; 
    Ang_Fall_F = [-1.0, 0, 10, 25, 40, 55, 75, 85, 89, 90, 90.1, 90.2];
    
    if theta_f_des >= last_theta_f
        FAV = interp1(Ang_Rise_F, I_axis_F, theta_f_des, 'linear', 'extrap');
    else
        FAV = interp1(Ang_Fall_F, I_axis_F, theta_f_des, 'linear', 'extrap');
    end
    FAV = max(0, min(350, FAV));
    
    % =====================================================================
    % 5. 状态更新
    % =====================================================================
    last_theta_p = theta_p_des;
    last_theta_f = theta_f_des;

end

== matlab function AirManagementSystem/Engine Bleed Air System/Precooler/LoadValueFlow ==
  data: X31 input; W_load output; X32 input; BPS input; BTS input
function W_load = LoadValueFlow(X31, X32, BPS, BTS)
    % =========================================================================
    % LoadValveFlow: 下游双管路负载流量计算模块
    %
    % --- 修正说明 ---
    % 1. 修复了温度计算错误：输入的 BTS 是摄氏度，必须转为开尔文计算流量。
    % 2. 修正了注释，明确需要 4 个输入。
    %
    % --- 输入 (Inputs) ---
    % 1. X31    : 下游管路31空调路 阀门开度指令 [%] (0~100)
    % 2. X32    : 下游管路32防冰路 阀门开度指令 [%] (0~100)
    % 3. BPS    : 上游压力 (即 Precooler 输出的 BPS) [kPa]
    % 4. BTS    : 上游温度 (即 Precooler 输出的 BTS) [degC]
    %
    % --- 输出 (Outputs) ---
    % 1. W_load : 总排气流量 [kg/h]
    % =========================================================================

    % --- 物理常数 ---
    R = 287.05;       
    Gamma = 1.4;      
    P_amb_Pa = 101325; 
    
    % --- 单位转换 ---
    Pup_load = BPS * 1000;        % [kPa] -> [Pa]
    T_up_K   = BTS + 273.15;      % [degC] -> [K]
    
    % --- 计算总流通面积 ---
    D_load = 0.1;   % DN100 [m]
    Cd_load = 0.8;  
    A_max_single = pi * D_load^2 / 4;

    ratio1 = max(min(X31, 100), 0) / 100;
    ratio2 = max(min(X32, 100), 0) / 100;
    
    A1 = Cd_load * A_max_single * ratio1;
    A2 = Cd_load * A_max_single * ratio2;
    A_load_total = A1 + A2;
    
    % --- 计算流量 ---
    Pdn_load = P_amb_Pa;     
    
    % 只有当上游压力大于环境压力，且阀门有开度时才计算
    % 增加 T_up_K > 0 保护，防止仿真初期温度异常导致 sqrt 报错
    if Pup_load > Pdn_load && A_load_total > 1e-6 && T_up_K > 0
        pr_load = Pdn_load / Pup_load;
        
        if pr_load < 0.528
            Psi_load = sqrt(Gamma * (2/(Gamma+1))^((Gamma+1)/(Gamma-1)));
        else
            Psi_load = sqrt(2*Gamma/(Gamma-1) * (pr_load^(2/Gamma) - pr_load^((Gamma+1)/Gamma)));
        end
        
        % 使用开尔文温度 T_up_K 进行计算
        W_load_kgs = A_load_total * (Pup_load / sqrt(R * T_up_K)) * Psi_load;
        
        W_load = W_load_kgs * 3600;
    else
        W_load = 0;
    end
end

== matlab function AirManagementSystem/Engine Bleed Air System/Precooler/Precooler ==
  data: W_load_in input; theta_PRSOV input; BPS output; theta_FAV input; P_comp input; BTS output; Q30 output; T_comp input; P_fan input; T_fan input; dt parameter
function [BPS, BTS, Q30] = Precooler(W_load_in, theta_PRSOV, theta_FAV, P_comp, T_comp, P_fan, T_fan, dt)
    % =========================================================================
    % Precooler Integrated Plant Model
    %
    % --- 输入 (Inputs) ---
    % 1. theta_PRSOV : 压力调节关断阀(PRSOV)开度角度 [deg] (0~90)
    % 2. T_comp      : 压气机引气温度 [degC]
    % 3. P_fan       : 风扇流路压力 [kPa]
    % 4. T_fan       : 风扇流路温度 [degC]
    % 5. theta_FAV   : 风扇空气阀(FAV)开度角度 [deg] (0~90)
    % 6. P_comp      : 压气机引气压力 [kPa]
    % 7. W_load_in   : 外部输入的下游负载流量 [kg/h] 
    %                  (由 LoadValveFlow 函数计算得出)
    %
    % --- 输出 (Outputs) ---
    % 1. BPS         : 预冷器热路出口压力 (Bleed Pressure Sensor) [kPa]
    % 2. BTS         : 预冷器热路出口温度 (Bleed Temperature Sensor) [degC]
    % 3. Q30         : 预冷器热路出口引气流量 [kg/h]
    % =========================================================================

    % --- 状态变量声明 ---
    % P_store: 下游管路容腔压力 [Pa]
    % T_store: 下游管路容腔温度 [K] (混合后的最终温度)
    % T_hx_out: 预冷器芯体出口温度 [K] (新增状态，体现换热器本身的热惯性)
    persistent P_store T_store T_hx_out
    
    % 物理常数
    R = 287.05;       
    Gamma = 1.4;      
    P_amb_Pa = 101325;
    
    % 下游容积计算
    % 2个管路，每个均为 DN100，长度 5m
    Vol = 2 * (pi * 0.05^2 * 5);          
    
    % --- 初始化 ---
    if isempty(P_store)
        P_store = P_amb_Pa;         % 初始为环境压力
        T_store = T_comp + 273.15;  % 初始温度
        T_hx_out = T_comp + 273.15; 
    end
    
    % 单位转换
    P_comp_Pa = P_comp * 1000;       
    T_comp_K  = T_comp + 273.15;
    P_fan_Pa  = P_fan * 1000;        
    T_fan_K   = T_fan + 273.15;        
    
    % =====================================================================
    % 1. 进气流量计算 (Source Flow)
    % =====================================================================
    
    % --- 热路入口阀 (PRSOV) ---
    D_prsov = 0.1;    
    Cd_prsov = 0.8;   
    phi_p = theta_PRSOV * (pi/180); 
    A_prsov = Cd_prsov * (pi * D_prsov^2 / 4) * (1 - cos(phi_p));
    
     % 判断流向
    if P_comp_Pa >= P_store
        Pup = P_comp_Pa; Pdn = P_store; T_up = T_comp_K; Is_Reverse = 1;
    else
        Pup = P_store; Pdn = P_comp_Pa; T_up = T_store; Is_Reverse = -1;
    end
    
    % 计算流量 (圣维南公式)
    if Pup > 1 && A_prsov > 1e-6
        pr = Pdn / Pup; 
        if pr > 1, pr = 1; end 
        if pr < 0, pr = 0; end

        pr_crit = 0.528; 
        if pr < pr_crit
            Psi = sqrt(Gamma * (2/(Gamma+1))^((Gamma+1)/(Gamma-1))); 
        else
            Psi = sqrt(2*Gamma/(Gamma-1) * (pr^(2/Gamma) - pr^((Gamma+1)/Gamma)));
        end
        W_bleed = A_prsov * (Pup / sqrt(R * T_up)) * Psi * Is_Reverse;
    else
        W_bleed = 0;
    end
    
    Q30 = W_bleed * 3600; 

    % =====================================================================
    % 2. 冷却气流计算 (Cooling Flow)
    % =====================================================================
    D_fav = 0.14;     
    Cd_fav = 0.8;     
    phi_f = theta_FAV * (pi/180);
    A_fav = Cd_fav * (pi * D_fav^2 / 4) * (1 - cos(phi_f));
    
    if P_fan_Pa > P_amb_Pa && A_fav > 0
        ratio = P_amb_Pa / P_fan_Pa;
        if ratio > 0.528
            Psi_f = sqrt(2*Gamma/((Gamma-1)*R*T_fan_K) * (ratio^(2/Gamma) - ratio^((Gamma+1)/Gamma)));
        else
            Psi_f = sqrt(2*Gamma/((Gamma-1)*R*T_fan_K) * (0.528^(2/Gamma) - 0.528^((Gamma+1)/Gamma)));
        end
        W_fan = A_fav * P_fan_Pa * Psi_f;
    else
        W_fan = 0;
    end
    
    % =====================================================================
    % 3. 换热机理修正
    % 参考文献[1]: 石周正, 等. 飞行器引气系统预冷器动态模型搭建及辨识研究[J]. 
    %          西北工业大学学报, 2024, 42(6): 1089-1098.
    %   1. 引入了论文中的"变时间常数"热惯性机理 (Eq. 14)。
    %   2. 将瞬态换热改为一阶动态响应过程，更符合物理实测。
    % =====================================================================
    
    % 3.1 计算稳态目标温度 (Steady State Target)
    % 这是假设时间无限长后应该达到的温度
    if abs(W_bleed) > 1e-4
        flow_ratio = W_fan / abs(W_bleed);
        
        % 效率曲线
        % 参考文献[2]: 卜绍志.飞机引气系统温度控制研究[J].内燃机与配件,2025,(13):52-54.
        x_d = [0, 0.26, 0.76, 1.26, 1.76, 2.26, 2.76, 3.26, 4.0, 5.0];
        y_d = [0, 0.32, 0.65, 0.78, 0.85, 0.89, 0.92, 0.94, 0.96, 0.97];
        
        % 限制输入范围，防止超出插值表
        flow_ratio_clamped = min(max(flow_ratio, 0), 5.0);
        eta = interp1(x_d, y_d, flow_ratio_clamped, 'linear');
        
        T_target = T_comp_K - eta * (T_comp_K - T_fan_K);
        
        
        % 3.2 计算流速与时间常数 (参考文献[1] Eq. 14)
        % 估算流经预冷器芯体的热路流速 v_h [m/s]
        % 假设芯体有效流通面积 A_core (需根据预冷器尺寸估算，例如 0.005 m^2)
        A_core = 0.005; 
        % 密度 rho = P / (R * T)
        rho_h = Pup / (R * T_up);
        v_h = abs(W_bleed) / (rho_h * A_core);
        
        % 防止 v_h 过小导致除零或时间常数过大
        v_h = max(v_h, 0.5); 
        
        % 参考文献[1] Eq. 14: tau = 38.02 * v^(-0.394)
        % 系数 38.02 是论文针对特定型号辨识的，可作为通用参考
        tau_hx = 38.02 * (v_h ^ -0.394);
        
        % 限制时间常数范围 (例如 0.1s 到 10s)
        tau_hx = max(min(tau_hx, 10), 0.1);
        
        % 2.3 换热器热惯性动态更新 (一阶滞后)
        % dT_hx/dt = (T_target - T_hx_out) / tau
        dT_hx = (T_target - T_hx_out) / tau_hx * dt;
        T_hx_out = T_hx_out + dT_hx;
        
    else
        % 无流量时，温度趋向于环境或保持不变
        % 这里简化为缓慢趋向于环境温度 (自然冷却)
        tau_cooling = 20.0; % 较慢的自然冷却
        dT_hx = (T_comp_K - T_hx_out) / tau_cooling * dt; 
        T_hx_out = T_hx_out + dT_hx;
    end
    
    % =====================================================================
    % 4. 容腔动态积分 (Chamber Integration)
    % =====================================================================
    
    % 直接使用外部输入的 W_load_in
    % W_load_in 必须为正值 (流出)
    % 输入单位是 [kg/h]，物理计算需要 [kg/s]，所以除以 3600
    W_load = abs(W_load_in) / 3600.0;
    
    % 4.1 压力积分
    dP = (R * T_store / Vol) * (W_bleed - W_load) * dt;

    P_new = P_store + dP;
    if P_new < P_amb_Pa
        P_new = P_amb_Pa;
    end
    
    % 4.2 温度积分
    Current_Mass = P_store * Vol / (R * T_store);
    if Current_Mass < 1e-4; Current_Mass = 1e-4; end
    
    if W_bleed > 0
        % 正向流：T_hx_out 进入容腔与 T_store 混合
        dT_chamber = (1/Current_Mass) * (W_bleed * (T_hx_out - T_store)) * dt;
    else
        % 反向流或无流：温度缓慢恢复到环境或保持
        dT_chamber = -0.01 * (T_store - 293.15) * dt;
    end
    
    T_new = T_store + dT_chamber;
    
    % 更新状态
    P_store = P_new;
    T_store = T_new;
    
    % 输出赋值
    BPS = P_store / 1000;           
    BTS = T_store - 273.15;   
end
